simulink model "FFM_Punch"  (R2017a)
settings: Solver=ode3  StartTime=0.0  StopTime=timesteps  FixedStep=data.SIM.Ts  RelTol=1e-3  EnableMultiTasking=on
values from neighbouring files (symbols this model uses):
  data =     [dakota_config.mat]
  downshift_map = data.TCU.upshift.veh_spd_default    [Simulation_results.m]
  upshift_map = data.TCU.upshift.veh_spd_default    [Simulation_results.m]
undefined symbols (not defined in the file or in its folder): air_density, Cd, DiscIntNeverNeededParam, fr_crankshaft, fr_speed_values, g, i_FD, ICE, Low_Ratio, M_Eng_Max, M_Eng_Max_Max, M_Eng_Max_Rpm, mt2m_f, mu_Roll_C0, mu_Roll_C1, mu_Roll_C2, Mv, n_Idle_Eng, Overdrive_Ratio, Re, S_eff_drag, Ts
(part 2 of 15)

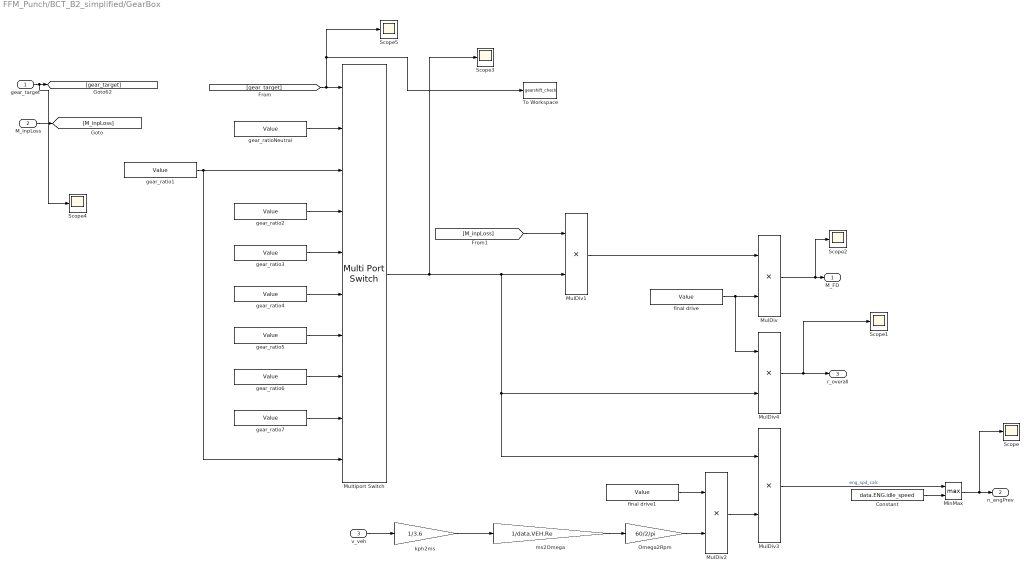
== system FFM_Punch/BCT_B2_simplified/GearBox ==
  gear_target : Inport
  M_inpLoss : Inport  Port=2
  v_veh : Inport  Port=3
  Constant : Constant  Value=data.ENG.idle_speed  OutDataTypeStr=single
  MinMax : MinMax  Function=max  Inputs=2  InputSameDT=on
  MulDiv : Product  Tag=Controls_Lib  Description=MulDiv  Inputs=**  CollapseDim=CollapseDim  OutMin=OutMin  OutMax=OutMax  OutDataTypeStr=single  SampleTime=SampleTime  InputSameDT=on  mask(MulDiv){Inputs=**, Multiplication=Element-wise(.*), CollapseMode=All dimensions, CollapseDim=1, SampleTime=-1, InputSameDT=on, OutMin=[], OutMax=[], OutDataTypeStr=single, LockScale=off, RndMeth=Floor, SaturateOnIntegerOverflow=off}
      mask prompts: Inputs "Number of inputs:"; CollapseMode "Multiply over:"; CollapseDim "Dimension:"; SampleTime "Sample time (-1 for inherited):"; InputSameDT "Require all inputs to have the same data type"; OutMin "Output minimum:"; OutMax "Output maximum:"; OutDataTypeStr "Output data type:"; LockScale "Lock output data type setting against changes by the fixed-point tools"; RndMeth "Integer rounding mode:"; SaturateOnIntegerOverflow "Saturate on integer overflow"
      mask help:
      | Multiply or divide inputs element-wise. Specify one of the following:
      |  a) * or / for each input port. For example, **/* performs the operation 'u1*u2/u3*u4'.
      |  b) scalar specifies the number of input ports to be multiplied.
      | If there is only one input port and the Multiplication parameter is set to Element-wise(.*), a single * or / collapses the input signal using the specified operation.
      mask Help: web([fileparts(which('Lib_built')) filesep 'hlp' filesep 'lib_MulDiv' '.html'], '-helpbrowser')
      mask TypeOptions Inputs: Inputs
      mask TypeOptions Multiplication: Multiplication
      mask TypeOptions CollapseMode: CollapseMode
      mask TypeOptions CollapseDim: CollapseDim
      mask TypeOptions SampleTime: SampleTime
      mask TypeOptions InputSameDT: InputSameDT
      mask TypeOptions OutMin: OutMin
      mask TypeOptions OutMax: OutMax
      mask TypeOptions OutDataTypeStr: OutDataTypeStr
      mask TypeOptions LockScale: LockScale
      mask TypeOptions RndMeth: RndMeth
      mask TypeOptions SaturateOnIntegerOverflow: SaturateOnIntegerOverflow
  MulDiv1 : Product  Tag=Controls_Lib  Description=MulDiv  Inputs=**  CollapseDim=CollapseDim  OutMin=OutMin  OutMax=OutMax  OutDataTypeStr=single  SampleTime=SampleTime  InputSameDT=on  mask(MulDiv){Inputs=**, Multiplication=Element-wise(.*), CollapseMode=All dimensions, CollapseDim=1, SampleTime=-1, InputSameDT=on, OutMin=[], OutMax=[], OutDataTypeStr=single, LockScale=off, RndMeth=Floor, SaturateOnIntegerOverflow=off}
      mask prompts: Inputs "Number of inputs:"; CollapseMode "Multiply over:"; CollapseDim "Dimension:"; SampleTime "Sample time (-1 for inherited):"; InputSameDT "Require all inputs to have the same data type"; OutMin "Output minimum:"; OutMax "Output maximum:"; OutDataTypeStr "Output data type:"; LockScale "Lock output data type setting against changes by the fixed-point tools"; RndMeth "Integer rounding mode:"; SaturateOnIntegerOverflow "Saturate on integer overflow"
      mask help:
      | Multiply or divide inputs element-wise. Specify one of the following:
      |  a) * or / for each input port. For example, **/* performs the operation 'u1*u2/u3*u4'.
      |  b) scalar specifies the number of input ports to be multiplied.
      | If there is only one input port and the Multiplication parameter is set to Element-wise(.*), a single * or / collapses the input signal using the specified operation.
      mask Help: web([fileparts(which('Lib_built')) filesep 'hlp' filesep 'lib_MulDiv' '.html'], '-helpbrowser')
      mask TypeOptions Inputs: Inputs
      mask TypeOptions Multiplication: Multiplication
      mask TypeOptions CollapseMode: CollapseMode
      mask TypeOptions CollapseDim: CollapseDim
      mask TypeOptions SampleTime: SampleTime
      mask TypeOptions InputSameDT: InputSameDT
      mask TypeOptions OutMin: OutMin
      mask TypeOptions OutMax: OutMax
      mask TypeOptions OutDataTypeStr: OutDataTypeStr
      mask TypeOptions LockScale: LockScale
      mask TypeOptions RndMeth: RndMeth
      mask TypeOptions SaturateOnIntegerOverflow: SaturateOnIntegerOverflow
  MulDiv2 : Product  Tag=Controls_Lib  Description=MulDiv  Inputs=**  CollapseDim=CollapseDim  OutMin=OutMin  OutMax=OutMax  OutDataTypeStr=single  SampleTime=SampleTime  InputSameDT=on  mask(MulDiv){Inputs=**, Multiplication=Element-wise(.*), CollapseMode=All dimensions, CollapseDim=1, SampleTime=-1, InputSameDT=on, OutMin=[], OutMax=[], OutDataTypeStr=single, LockScale=off, RndMeth=Floor, SaturateOnIntegerOverflow=off}
      mask prompts: Inputs "Number of inputs:"; CollapseMode "Multiply over:"; CollapseDim "Dimension:"; SampleTime "Sample time (-1 for inherited):"; InputSameDT "Require all inputs to have the same data type"; OutMin "Output minimum:"; OutMax "Output maximum:"; OutDataTypeStr "Output data type:"; LockScale "Lock output data type setting against changes by the fixed-point tools"; RndMeth "Integer rounding mode:"; SaturateOnIntegerOverflow "Saturate on integer overflow"
      mask help:
      | Multiply or divide inputs element-wise. Specify one of the following:
      |  a) * or / for each input port. For example, **/* performs the operation 'u1*u2/u3*u4'.
      |  b) scalar specifies the number of input ports to be multiplied.
      | If there is only one input port and the Multiplication parameter is set to Element-wise(.*), a single * or / collapses the input signal using the specified operation.
      mask Help: web([fileparts(which('Lib_built')) filesep 'hlp' filesep 'lib_MulDiv' '.html'], '-helpbrowser')
      mask TypeOptions Inputs: Inputs
      mask TypeOptions Multiplication: Multiplication
      mask TypeOptions CollapseMode: CollapseMode
      mask TypeOptions CollapseDim: CollapseDim
      mask TypeOptions SampleTime: SampleTime
      mask TypeOptions InputSameDT: InputSameDT
      mask TypeOptions OutMin: OutMin
      mask TypeOptions OutMax: OutMax
      mask TypeOptions OutDataTypeStr: OutDataTypeStr
      mask TypeOptions LockScale: LockScale
      mask TypeOptions RndMeth: RndMeth
      mask TypeOptions SaturateOnIntegerOverflow: SaturateOnIntegerOverflow
  MulDiv3 : Product  Tag=Controls_Lib  Description=MulDiv  Inputs=**  CollapseDim=CollapseDim  OutMin=OutMin  OutMax=OutMax  OutDataTypeStr=single  SampleTime=SampleTime  InputSameDT=on  mask(MulDiv){Inputs=**, Multiplication=Element-wise(.*), CollapseMode=All dimensions, CollapseDim=1, SampleTime=-1, InputSameDT=on, OutMin=[], OutMax=[], OutDataTypeStr=single, LockScale=off, RndMeth=Floor, SaturateOnIntegerOverflow=off}
      mask prompts: Inputs "Number of inputs:"; CollapseMode "Multiply over:"; CollapseDim "Dimension:"; SampleTime "Sample time (-1 for inherited):"; InputSameDT "Require all inputs to have the same data type"; OutMin "Output minimum:"; OutMax "Output maximum:"; OutDataTypeStr "Output data type:"; LockScale "Lock output data type setting against changes by the fixed-point tools"; RndMeth "Integer rounding mode:"; SaturateOnIntegerOverflow "Saturate on integer overflow"
      mask help:
      | Multiply or divide inputs element-wise. Specify one of the following:
      |  a) * or / for each input port. For example, **/* performs the operation 'u1*u2/u3*u4'.
      |  b) scalar specifies the number of input ports to be multiplied.
      | If there is only one input port and the Multiplication parameter is set to Element-wise(.*), a single * or / collapses the input signal using the specified operation.
      mask Help: web([fileparts(which('Lib_built')) filesep 'hlp' filesep 'lib_MulDiv' '.html'], '-helpbrowser')
      mask TypeOptions Inputs: Inputs
      mask TypeOptions Multiplication: Multiplication
      mask TypeOptions CollapseMode: CollapseMode
      mask TypeOptions CollapseDim: CollapseDim
      mask TypeOptions SampleTime: SampleTime
      mask TypeOptions InputSameDT: InputSameDT
      mask TypeOptions OutMin: OutMin
      mask TypeOptions OutMax: OutMax
      mask TypeOptions OutDataTypeStr: OutDataTypeStr
      mask TypeOptions LockScale: LockScale
      mask TypeOptions RndMeth: RndMeth
      mask TypeOptions SaturateOnIntegerOverflow: SaturateOnIntegerOverflow
  MulDiv4 : Product  Tag=Controls_Lib  Description=MulDiv  Inputs=**  CollapseDim=CollapseDim  OutMin=OutMin  OutMax=OutMax  OutDataTypeStr=single  SampleTime=SampleTime  InputSameDT=on  mask(MulDiv){Inputs=**, Multiplication=Element-wise(.*), CollapseMode=All dimensions, CollapseDim=1, SampleTime=-1, InputSameDT=on, OutMin=[], OutMax=[], OutDataTypeStr=single, LockScale=off, RndMeth=Floor, SaturateOnIntegerOverflow=off}
      mask prompts: Inputs "Number of inputs:"; CollapseMode "Multiply over:"; CollapseDim "Dimension:"; SampleTime "Sample time (-1 for inherited):"; InputSameDT "Require all inputs to have the same data type"; OutMin "Output minimum:"; OutMax "Output maximum:"; OutDataTypeStr "Output data type:"; LockScale "Lock output data type setting against changes by the fixed-point tools"; RndMeth "Integer rounding mode:"; SaturateOnIntegerOverflow "Saturate on integer overflow"
      mask help:
      | Multiply or divide inputs element-wise. Specify one of the following:
      |  a) * or / for each input port. For example, **/* performs the operation 'u1*u2/u3*u4'.
      |  b) scalar specifies the number of input ports to be multiplied.
      | If there is only one input port and the Multiplication parameter is set to Element-wise(.*), a single * or / collapses the input signal using the specified operation.
      mask Help: web([fileparts(which('Lib_built')) filesep 'hlp' filesep 'lib_MulDiv' '.html'], '-helpbrowser')
      mask TypeOptions Inputs: Inputs
      mask TypeOptions Multiplication: Multiplication
      mask TypeOptions CollapseMode: CollapseMode
      mask TypeOptions CollapseDim: CollapseDim
      mask TypeOptions SampleTime: SampleTime
      mask TypeOptions InputSameDT: InputSameDT
      mask TypeOptions OutMin: OutMin
      mask TypeOptions OutMax: OutMax
      mask TypeOptions OutDataTypeStr: OutDataTypeStr
      mask TypeOptions LockScale: LockScale
      mask TypeOptions RndMeth: RndMeth
      mask TypeOptions SaturateOnIntegerOverflow: SaturateOnIntegerOverflow
  Multiport Switch : MultiPortSwitch  DataPortOrder=Specify indices  DataPortIndices={0,1,2,3,4,5,6,7}  DataPortForDefault=Additional data port  DiagnosticForDefault=None
  Omega2Rpm : Gain  Gain=60/2/pi
  Scope{,1..5} (6 alike) : Scope
  To Workspace : ToWorkspace  VariableName=gearshift_check  SampleTime=-1
  final drive : Constant  Tag=Controls_Lib  Description=constant  Value=Value  OutMin=OutMin  OutMax=OutMax  OutDataTypeStr=Inherit: Inherit via back propagation  SampleTime=SampleTime  FramePeriod=FramePeriod  mask(Constant){Value=data.DCT.ratio.r_fd, VectorParams1D=on, SampleTime=-1, FramePeriod=inf, OutMin=[], OutMax=[], OutDataTypeStr=Inherit: Inherit via back propagation, LockScale=off}
      mask prompts: Value "Simulink:blkprm_prompts:ConstConstValue"; VectorParams1D "Simulink:blkprm_prompts:AllSrcsVector1D"; SampleTime "Simulink:blkprm_prompts:AllSrcBlksSampleTime"; FramePeriod "Simulink:blkprm_prompts:AllSrcBlksFramePeriod"; OutMin "Simulink:blkprm_prompts:OutputDesignMin"; OutMax "Simulink:blkprm_prompts:OutputDesignMax"; OutDataTypeStr "Simulink:blkprm_prompts:OUTPUT_UNIFIEDDATATYPE"; LockScale "Simulink:blkprm_prompts:LockScale"
      mask help: Output the constant specified by the 'Constant value' parameter.
      mask Help: web([fileparts(which('Lib_built')) filesep 'hlp' filesep 'lib_constant' '.html'], '-helpbrowser')
      mask TypeOptions Value: Value
      mask TypeOptions VectorParams1D: VectorParams1D
      mask TypeOptions SampleTime: SampleTime
      mask TypeOptions FramePeriod: FramePeriod
      mask TypeOptions OutMin: OutMin
      mask TypeOptions OutMax: OutMax
      mask TypeOptions OutDataTypeStr: OutDataTypeStr
      mask TypeOptions LockScale: LockScale
      mask DialogControl ParameterTabVar0 Prompt: Main
      mask Display: disp(get_param(gcb,'Value'))
  final drive1 : Constant  Tag=Controls_Lib  Description=constant  Value=Value  OutMin=OutMin  OutMax=OutMax  OutDataTypeStr=Inherit: Inherit via back propagation  SampleTime=SampleTime  FramePeriod=FramePeriod  mask(Constant){Value=data.DCT.ratio.r_fd, VectorParams1D=on, SampleTime=-1, FramePeriod=inf, OutMin=[], OutMax=[], OutDataTypeStr=Inherit: Inherit via back propagation, LockScale=off}
      mask prompts: Value "Simulink:blkprm_prompts:ConstConstValue"; VectorParams1D "Simulink:blkprm_prompts:AllSrcsVector1D"; SampleTime "Simulink:blkprm_prompts:AllSrcBlksSampleTime"; FramePeriod "Simulink:blkprm_prompts:AllSrcBlksFramePeriod"; OutMin "Simulink:blkprm_prompts:OutputDesignMin"; OutMax "Simulink:blkprm_prompts:OutputDesignMax"; OutDataTypeStr "Simulink:blkprm_prompts:OUTPUT_UNIFIEDDATATYPE"; LockScale "Simulink:blkprm_prompts:LockScale"
      mask help: Output the constant specified by the 'Constant value' parameter.
      mask Help: web([fileparts(which('Lib_built')) filesep 'hlp' filesep 'lib_constant' '.html'], '-helpbrowser')
      mask TypeOptions Value: Value
      mask TypeOptions VectorParams1D: VectorParams1D
      mask TypeOptions SampleTime: SampleTime
      mask TypeOptions FramePeriod: FramePeriod
      mask TypeOptions OutMin: OutMin
      mask TypeOptions OutMax: OutMax
      mask TypeOptions OutDataTypeStr: OutDataTypeStr
      mask TypeOptions LockScale: LockScale
      mask DialogControl ParameterTabVar0 Prompt: Main
      mask Display: disp(get_param(gcb,'Value'))
  gear_ratio1 : Constant  Tag=Controls_Lib  Description=constant  Value=Value  OutMin=OutMin  OutMax=OutMax  OutDataTypeStr=Inherit: Inherit via back propagation  SampleTime=SampleTime  FramePeriod=FramePeriod  mask(Constant){Value=data.DCT.ratio.r_1_C, VectorParams1D=on, SampleTime=-1, FramePeriod=inf, OutMin=[], OutMax=[], OutDataTypeStr=Inherit: Inherit via back propagation, LockScale=off}
      mask prompts: Value "Simulink:blkprm_prompts:ConstConstValue"; VectorParams1D "Simulink:blkprm_prompts:AllSrcsVector1D"; SampleTime "Simulink:blkprm_prompts:AllSrcBlksSampleTime"; FramePeriod "Simulink:blkprm_prompts:AllSrcBlksFramePeriod"; OutMin "Simulink:blkprm_prompts:OutputDesignMin"; OutMax "Simulink:blkprm_prompts:OutputDesignMax"; OutDataTypeStr "Simulink:blkprm_prompts:OUTPUT_UNIFIEDDATATYPE"; LockScale "Simulink:blkprm_prompts:LockScale"
      mask help: Output the constant specified by the 'Constant value' parameter.
      mask Help: web([fileparts(which('Lib_built')) filesep 'hlp' filesep 'lib_constant' '.html'], '-helpbrowser')
      mask TypeOptions Value: Value
      mask TypeOptions VectorParams1D: VectorParams1D
      mask TypeOptions SampleTime: SampleTime
      mask TypeOptions FramePeriod: FramePeriod
      mask TypeOptions OutMin: OutMin
      mask TypeOptions OutMax: OutMax
      mask TypeOptions OutDataTypeStr: OutDataTypeStr
      mask TypeOptions LockScale: LockScale
      mask DialogControl ParameterTabVar0 Prompt: Main
      mask Display: disp(get_param(gcb,'Value'))
  gear_ratio2 : Constant  Tag=Controls_Lib  Description=constant  Value=Value  OutMin=OutMin  OutMax=OutMax  OutDataTypeStr=Inherit: Inherit via back propagation  SampleTime=SampleTime  FramePeriod=FramePeriod  mask(Constant){Value=data.DCT.ratio.r_2_C, VectorParams1D=on, SampleTime=-1, FramePeriod=inf, OutMin=[], OutMax=[], OutDataTypeStr=Inherit: Inherit via back propagation, LockScale=off}
      mask prompts: Value "Simulink:blkprm_prompts:ConstConstValue"; VectorParams1D "Simulink:blkprm_prompts:AllSrcsVector1D"; SampleTime "Simulink:blkprm_prompts:AllSrcBlksSampleTime"; FramePeriod "Simulink:blkprm_prompts:AllSrcBlksFramePeriod"; OutMin "Simulink:blkprm_prompts:OutputDesignMin"; OutMax "Simulink:blkprm_prompts:OutputDesignMax"; OutDataTypeStr "Simulink:blkprm_prompts:OUTPUT_UNIFIEDDATATYPE"; LockScale "Simulink:blkprm_prompts:LockScale"
      mask help: Output the constant specified by the 'Constant value' parameter.
      mask Help: web([fileparts(which('Lib_built')) filesep 'hlp' filesep 'lib_constant' '.html'], '-helpbrowser')
      mask TypeOptions Value: Value
      mask TypeOptions VectorParams1D: VectorParams1D
      mask TypeOptions SampleTime: SampleTime
      mask TypeOptions FramePeriod: FramePeriod
      mask TypeOptions OutMin: OutMin
      mask TypeOptions OutMax: OutMax
      mask TypeOptions OutDataTypeStr: OutDataTypeStr
      mask TypeOptions LockScale: LockScale
      mask DialogControl ParameterTabVar0 Prompt: Main
      mask Display: disp(get_param(gcb,'Value'))
  gear_ratio3 : Constant  Tag=Controls_Lib  Description=constant  Value=Value  OutMin=OutMin  OutMax=OutMax  OutDataTypeStr=Inherit: Inherit via back propagation  SampleTime=SampleTime  FramePeriod=FramePeriod  mask(Constant){Value=data.DCT.ratio.r_3_C, VectorParams1D=on, SampleTime=-1, FramePeriod=inf, OutMin=[], OutMax=[], OutDataTypeStr=Inherit: Inherit via back propagation, LockScale=off}
      mask prompts: Value "Simulink:blkprm_prompts:ConstConstValue"; VectorParams1D "Simulink:blkprm_prompts:AllSrcsVector1D"; SampleTime "Simulink:blkprm_prompts:AllSrcBlksSampleTime"; FramePeriod "Simulink:blkprm_prompts:AllSrcBlksFramePeriod"; OutMin "Simulink:blkprm_prompts:OutputDesignMin"; OutMax "Simulink:blkprm_prompts:OutputDesignMax"; OutDataTypeStr "Simulink:blkprm_prompts:OUTPUT_UNIFIEDDATATYPE"; LockScale "Simulink:blkprm_prompts:LockScale"
      mask help: Output the constant specified by the 'Constant value' parameter.
      mask Help: web([fileparts(which('Lib_built')) filesep 'hlp' filesep 'lib_constant' '.html'], '-helpbrowser')
      mask TypeOptions Value: Value
      mask TypeOptions VectorParams1D: VectorParams1D
      mask TypeOptions SampleTime: SampleTime
      mask TypeOptions FramePeriod: FramePeriod
      mask TypeOptions OutMin: OutMin
      mask TypeOptions OutMax: OutMax
      mask TypeOptions OutDataTypeStr: OutDataTypeStr
      mask TypeOptions LockScale: LockScale
      mask DialogControl ParameterTabVar0 Prompt: Main
      mask Display: disp(get_param(gcb,'Value'))
  gear_ratio4 : Constant  Tag=Controls_Lib  Description=constant  Value=Value  OutMin=OutMin  OutMax=OutMax  OutDataTypeStr=Inherit: Inherit via back propagation  SampleTime=SampleTime  FramePeriod=FramePeriod  mask(Constant){Value=data.DCT.ratio.r_4_C, VectorParams1D=on, SampleTime=-1, FramePeriod=inf, OutMin=[], OutMax=[], OutDataTypeStr=Inherit: Inherit via back propagation, LockScale=off}
      mask prompts: Value "Simulink:blkprm_prompts:ConstConstValue"; VectorParams1D "Simulink:blkprm_prompts:AllSrcsVector1D"; SampleTime "Simulink:blkprm_prompts:AllSrcBlksSampleTime"; FramePeriod "Simulink:blkprm_prompts:AllSrcBlksFramePeriod"; OutMin "Simulink:blkprm_prompts:OutputDesignMin"; OutMax "Simulink:blkprm_prompts:OutputDesignMax"; OutDataTypeStr "Simulink:blkprm_prompts:OUTPUT_UNIFIEDDATATYPE"; LockScale "Simulink:blkprm_prompts:LockScale"
      mask help: Output the constant specified by the 'Constant value' parameter.
      mask Help: web([fileparts(which('Lib_built')) filesep 'hlp' filesep 'lib_constant' '.html'], '-helpbrowser')
      mask TypeOptions Value: Value
      mask TypeOptions VectorParams1D: VectorParams1D
      mask TypeOptions SampleTime: SampleTime
      mask TypeOptions FramePeriod: FramePeriod
      mask TypeOptions OutMin: OutMin
      mask TypeOptions OutMax: OutMax
      mask TypeOptions OutDataTypeStr: OutDataTypeStr
      mask TypeOptions LockScale: LockScale
      mask DialogControl ParameterTabVar0 Prompt: Main
      mask Display: disp(get_param(gcb,'Value'))
  gear_ratio5 : Constant  Tag=Controls_Lib  Description=constant  Value=Value  OutMin=OutMin  OutMax=OutMax  OutDataTypeStr=Inherit: Inherit via back propagation  SampleTime=SampleTime  FramePeriod=FramePeriod  mask(Constant){Value=data.DCT.ratio.r_5_C, VectorParams1D=on, SampleTime=-1, FramePeriod=inf, OutMin=[], OutMax=[], OutDataTypeStr=Inherit: Inherit via back propagation, LockScale=off}
      mask prompts: Value "Simulink:blkprm_prompts:ConstConstValue"; VectorParams1D "Simulink:blkprm_prompts:AllSrcsVector1D"; SampleTime "Simulink:blkprm_prompts:AllSrcBlksSampleTime"; FramePeriod "Simulink:blkprm_prompts:AllSrcBlksFramePeriod"; OutMin "Simulink:blkprm_prompts:OutputDesignMin"; OutMax "Simulink:blkprm_prompts:OutputDesignMax"; OutDataTypeStr "Simulink:blkprm_prompts:OUTPUT_UNIFIEDDATATYPE"; LockScale "Simulink:blkprm_prompts:LockScale"
      mask help: Output the constant specified by the 'Constant value' parameter.
      mask Help: web([fileparts(which('Lib_built')) filesep 'hlp' filesep 'lib_constant' '.html'], '-helpbrowser')
      mask TypeOptions Value: Value
      mask TypeOptions VectorParams1D: VectorParams1D
      mask TypeOptions SampleTime: SampleTime
      mask TypeOptions FramePeriod: FramePeriod
      mask TypeOptions OutMin: OutMin
      mask TypeOptions OutMax: OutMax
      mask TypeOptions OutDataTypeStr: OutDataTypeStr
      mask TypeOptions LockScale: LockScale
      mask DialogControl ParameterTabVar0 Prompt: Main
      mask Display: disp(get_param(gcb,'Value'))
  gear_ratio6 : Constant  Tag=Controls_Lib  Description=constant  Value=Value  OutMin=OutMin  OutMax=OutMax  OutDataTypeStr=Inherit: Inherit via back propagation  SampleTime=SampleTime  FramePeriod=FramePeriod  mask(Constant){Value=data.DCT.ratio.r_6_C, VectorParams1D=on, SampleTime=-1, FramePeriod=inf, OutMin=[], OutMax=[], OutDataTypeStr=Inherit: Inherit via back propagation, LockScale=off}
      mask prompts: Value "Simulink:blkprm_prompts:ConstConstValue"; VectorParams1D "Simulink:blkprm_prompts:AllSrcsVector1D"; SampleTime "Simulink:blkprm_prompts:AllSrcBlksSampleTime"; FramePeriod "Simulink:blkprm_prompts:AllSrcBlksFramePeriod"; OutMin "Simulink:blkprm_prompts:OutputDesignMin"; OutMax "Simulink:blkprm_prompts:OutputDesignMax"; OutDataTypeStr "Simulink:blkprm_prompts:OUTPUT_UNIFIEDDATATYPE"; LockScale "Simulink:blkprm_prompts:LockScale"
      mask help: Output the constant specified by the 'Constant value' parameter.
      mask Help: web([fileparts(which('Lib_built')) filesep 'hlp' filesep 'lib_constant' '.html'], '-helpbrowser')
      mask TypeOptions Value: Value
      mask TypeOptions VectorParams1D: VectorParams1D
      mask TypeOptions SampleTime: SampleTime
      mask TypeOptions FramePeriod: FramePeriod
      mask TypeOptions OutMin: OutMin
      mask TypeOptions OutMax: OutMax
      mask TypeOptions OutDataTypeStr: OutDataTypeStr
      mask TypeOptions LockScale: LockScale
      mask DialogControl ParameterTabVar0 Prompt: Main
      mask Display: disp(get_param(gcb,'Value'))
  gear_ratio7 : Constant  Tag=Controls_Lib  Description=constant  Value=Value  OutMin=OutMin  OutMax=OutMax  OutDataTypeStr=Inherit: Inherit via back propagation  SampleTime=SampleTime  FramePeriod=FramePeriod  mask(Constant){Value=data.DCT.ratio.r_7_C, VectorParams1D=on, SampleTime=-1, FramePeriod=inf, OutMin=[], OutMax=[], OutDataTypeStr=Inherit: Inherit via back propagation, LockScale=off}
      mask prompts: Value "Simulink:blkprm_prompts:ConstConstValue"; VectorParams1D "Simulink:blkprm_prompts:AllSrcsVector1D"; SampleTime "Simulink:blkprm_prompts:AllSrcBlksSampleTime"; FramePeriod "Simulink:blkprm_prompts:AllSrcBlksFramePeriod"; OutMin "Simulink:blkprm_prompts:OutputDesignMin"; OutMax "Simulink:blkprm_prompts:OutputDesignMax"; OutDataTypeStr "Simulink:blkprm_prompts:OUTPUT_UNIFIEDDATATYPE"; LockScale "Simulink:blkprm_prompts:LockScale"
      mask help: Output the constant specified by the 'Constant value' parameter.
      mask Help: web([fileparts(which('Lib_built')) filesep 'hlp' filesep 'lib_constant' '.html'], '-helpbrowser')
      mask TypeOptions Value: Value
      mask TypeOptions VectorParams1D: VectorParams1D
      mask TypeOptions SampleTime: SampleTime
      mask TypeOptions FramePeriod: FramePeriod
      mask TypeOptions OutMin: OutMin
      mask TypeOptions OutMax: OutMax
      mask TypeOptions OutDataTypeStr: OutDataTypeStr
      mask TypeOptions LockScale: LockScale
      mask DialogControl ParameterTabVar0 Prompt: Main
      mask Display: disp(get_param(gcb,'Value'))
  gear_ratioNeutral : Constant  Tag=Controls_Lib  Description=constant  Value=Value  OutMin=OutMin  OutMax=OutMax  OutDataTypeStr=Inherit: Inherit via back propagation  SampleTime=SampleTime  FramePeriod=FramePeriod  mask(Constant){Value=0, VectorParams1D=on, SampleTime=-1, FramePeriod=inf, OutMin=[], OutMax=[], OutDataTypeStr=Inherit: Inherit via back propagation, LockScale=off}
      mask prompts: Value "Simulink:blkprm_prompts:ConstConstValue"; VectorParams1D "Simulink:blkprm_prompts:AllSrcsVector1D"; SampleTime "Simulink:blkprm_prompts:AllSrcBlksSampleTime"; FramePeriod "Simulink:blkprm_prompts:AllSrcBlksFramePeriod"; OutMin "Simulink:blkprm_prompts:OutputDesignMin"; OutMax "Simulink:blkprm_prompts:OutputDesignMax"; OutDataTypeStr "Simulink:blkprm_prompts:OUTPUT_UNIFIEDDATATYPE"; LockScale "Simulink:blkprm_prompts:LockScale"
      mask help: Output the constant specified by the 'Constant value' parameter.
      mask Help: web([fileparts(which('Lib_built')) filesep 'hlp' filesep 'lib_constant' '.html'], '-helpbrowser')
      mask TypeOptions Value: Value
      mask TypeOptions VectorParams1D: VectorParams1D
      mask TypeOptions SampleTime: SampleTime
      mask TypeOptions FramePeriod: FramePeriod
      mask TypeOptions OutMin: OutMin
      mask TypeOptions OutMax: OutMax
      mask TypeOptions OutDataTypeStr: OutDataTypeStr
      mask TypeOptions LockScale: LockScale
      mask DialogControl ParameterTabVar0 Prompt: Main
      mask Display: disp(get_param(gcb,'Value'))
  kph2ms : Gain  Gain=1/3.6
  ms2Omega : Gain  Gain=1/data.VEH.Re  OutDataTypeStr=Inherit: Inherit via back propagation  ParamDataTypeStr=Inherit: Same as input
  M_FD : Outport
  n_engPrev : Outport  Port=2
  r_overall : Outport  Port=3
  wires:
  MulDiv/1 -> Scope2/1, M_FD/1
  gear_target/1 -> Scope4/1, [gear_target]
  [gear_target] -> To Workspace/1, Scope5/1, Multiport Switch/1
  gear_ratio6/1 -> Multiport Switch/8
  gear_ratio5/1 -> Multiport Switch/7
  gear_ratio2/1 -> Multiport Switch/4
  gear_ratio7/1 -> Multiport Switch/9
  gear_ratio1/1 -> Multiport Switch/10, Multiport Switch/3
  gear_ratio4/1 -> Multiport Switch/6
  gear_ratioNeutral/1 -> Multiport Switch/2
  gear_ratio3/1 -> Multiport Switch/5
  M_inpLoss/1 -> [M_inpLoss]
  Multiport Switch/1 -> Scope3/1, MulDiv4/2, MulDiv3/1, MulDiv1/2
  [M_inpLoss] -> MulDiv1/1
  MulDiv1/1 -> MulDiv/1
  final drive/1 -> MulDiv4/1, MulDiv/2
  v_veh/1 -> kph2ms/1
  kph2ms/1 -> ms2Omega/1
  ms2Omega/1 -> Omega2Rpm/1
  Omega2Rpm/1 -> MulDiv2/2
  final drive1/1 -> MulDiv2/1
  MulDiv2/1 -> MulDiv3/2
  MulDiv4/1 -> Scope1/1, r_overall/1
  MulDiv3/1 -> MinMax/1  "eng_spd_calc"
  MinMax/1 -> Scope/1, n_engPrev/1
  Constant/1 -> MinMax/2

== system FFM_Punch/Controller/F02_03_03_03_Shift_Laws_Determination ==
  Throttle_pedal : Inport
  constant : Constant  Value=[1 2 3 4 5 6 7 8]  OutDataTypeStr=uint8
  constant1 : Constant  Value=[1 2 3 4 5 6 7 8]  OutDataTypeStr=uint8
  ts_v_autoModDownAdpLaw_M2 : Lookup_n-D  BreakpointsForDimension1=data.TCU.downshift.pedal  BreakpointsForDimension2=[1 2 3 4 5 6 7 8]  BreakpointsForDimension1DataTypeStr=single  BreakpointsForDimension2DataTypeStr=uint8  BeginIndexSearchUsingPreviousIndexResult=on  Table=downshift_map  TableDataTypeStr=single  ExtrapMethod=Clip  UseLastTableValue=on  InternalRulePriority=Speed  OutDataTypeStr=single  RndMeth=Simplest
      settings: AttributesFormatString=%<Table>
  ts_v_autoModUpAdpLaw_M2 : Lookup_n-D  BreakpointsForDimension1=data.TCU.upshift.pedal  BreakpointsForDimension2=[1 2 3 4 5 6 7 8]  BreakpointsForDimension1DataTypeStr=single  BreakpointsForDimension2DataTypeStr=uint8  BeginIndexSearchUsingPreviousIndexResult=on  Table=upshift_map  TableDataTypeStr=single  ExtrapMethod=Clip  UseLastTableValue=on  InternalRulePriority=Speed  OutDataTypeStr=single  RndMeth=Simplest
      settings: AttributesFormatString=%<Table>
  ts_v_vectThdAutoModDown : Outport
  ts_v_vectThdAutoModUp : Outport  Port=2
  wires:
  constant1/1 -> ts_v_autoModUpAdpLaw_M2/2
  [Throttle_pedal] -> ts_v_autoModDownAdpLaw_M2/1, ts_v_autoModUpAdpLaw_M2/1
  constant/1 -> ts_v_autoModDownAdpLaw_M2/2
  ts_v_autoModDownAdpLaw_M2/1 -> [ts_v_vectThdAutoModDown]
  ts_v_autoModUpAdpLaw_M2/1 -> [ts_v_vectThdAutoModUp]
  [ts_v_vectThdAutoModDown] -> ts_v_vectThdAutoModDown/1
  [ts_v_vectThdAutoModUp] -> ts_v_vectThdAutoModUp/1
  Throttle_pedal/1 -> [Throttle_pedal]

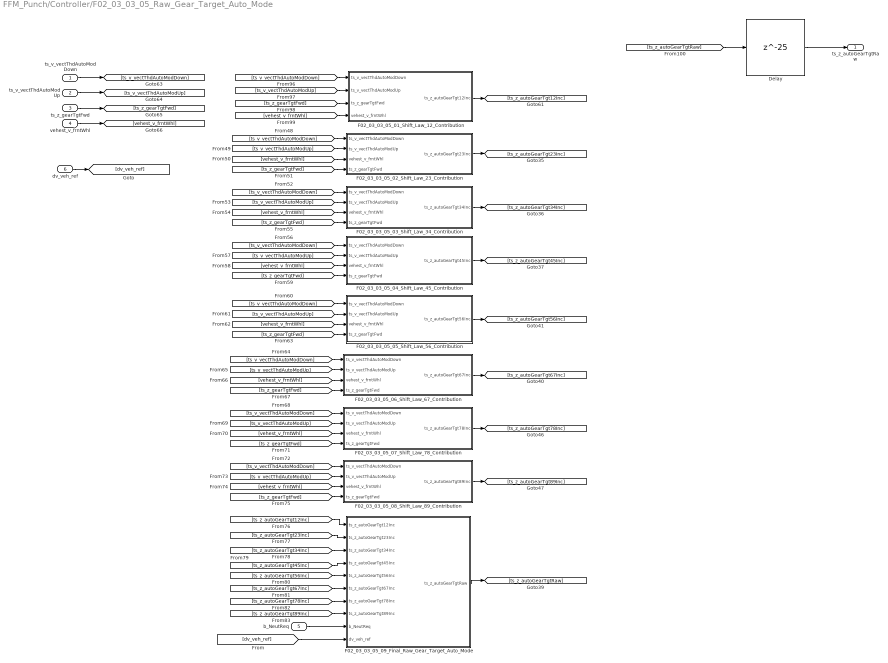
== system FFM_Punch/Controller/F02_03_03_05_Raw_Gear_Target_Auto_Mode ==
  ts_v_vectThdAutoModDown : Inport
  ts_v_vectThdAutoModUp : Inport  Port=2
  ts_z_gearTgtFwd : Inport  Port=3
  vehest_v_frntWhl : Inport  Port=4
  b_NeutReq : Inport  Port=5
  dv_veh_ref : Inport  Tag=Controls_Lib  Description=Inp  Port=6  Interpolate=off
  Delay : Delay  DelayLength=25  InitialCondition=1  UseCircularBuffer=on
  F02_03_03_05_01_Shift_Law_12_Contribution : Subsystem
  F02_03_03_05_02_Shift_Law_23_Contribution : Subsystem
  F02_03_03_05_03_Shift_Law_34_Contribution : Subsystem
  F02_03_03_05_04_Shift_Law_45_Contribution : Subsystem
  F02_03_03_05_05_Shift_Law_56_Contribution : Subsystem
  F02_03_03_05_06_Shift_Law_67_Contribution : Subsystem
  F02_03_03_05_07_Shift_Law_78_Contribution : Subsystem
  F02_03_03_05_08_Shift_Law_89_Contribution : Subsystem
  F02_03_03_05_09_Final_Raw_Gear_Target_Auto_Mode : Subsystem
  ts_z_autoGearTgtRaw : Outport
  wires:
  [ts_z_autoGearTgt89Inc] -> F02_03_03_05_09_Final_Raw_Gear_Target_Auto_Mode/8(ts_z_autoGearTgt89Inc)
  [ts_z_autoGearTgt78Inc] -> F02_03_03_05_09_Final_Raw_Gear_Target_Auto_Mode/7(ts_z_autoGearTgt78Inc)
  [ts_z_autoGearTgt67Inc] -> F02_03_03_05_09_Final_Raw_Gear_Target_Auto_Mode/6(ts_z_autoGearTgt67Inc)
  [ts_z_autoGearTgt56Inc] -> F02_03_03_05_09_Final_Raw_Gear_Target_Auto_Mode/5(ts_z_autoGearTgt56Inc)
  [ts_z_autoGearTgt45Inc] -> F02_03_03_05_09_Final_Raw_Gear_Target_Auto_Mode/4(ts_z_autoGearTgt45Inc)
  [ts_z_autoGearTgt34Inc] -> F02_03_03_05_09_Final_Raw_Gear_Target_Auto_Mode/3(ts_z_autoGearTgt34Inc)
  [ts_z_autoGearTgt23Inc] -> F02_03_03_05_09_Final_Raw_Gear_Target_Auto_Mode/2(ts_z_autoGearTgt23Inc)
  [ts_z_autoGearTgt12Inc] -> F02_03_03_05_09_Final_Raw_Gear_Target_Auto_Mode/1(ts_z_autoGearTgt12Inc)
  F02_03_03_05_08_Shift_Law_89_Contribution/1(ts_z_autoGearTgt89Inc) -> [ts_z_autoGearTgt89Inc]
  [ts_z_gearTgtFwd] -> F02_03_03_05_08_Shift_Law_89_Contribution/4(ts_z_gearTgtFwd)
  [vehest_v_frntWhl] -> F02_03_03_05_08_Shift_Law_89_Contribution/3(vehest_v_frntWhl)
  [ts_v_vectThdAutoModUp] -> F02_03_03_05_08_Shift_Law_89_Contribution/2(ts_v_vectThdAutoModUp)
  [ts_v_vectThdAutoModDown] -> F02_03_03_05_08_Shift_Law_89_Contribution/1(ts_v_vectThdAutoModDown)
  F02_03_03_05_07_Shift_Law_78_Contribution/1(ts_z_autoGearTgt78Inc) -> [ts_z_autoGearTgt78Inc]
  [ts_z_gearTgtFwd] -> F02_03_03_05_07_Shift_Law_78_Contribution/4(ts_z_gearTgtFwd)
  [vehest_v_frntWhl] -> F02_03_03_05_07_Shift_Law_78_Contribution/3(vehest_v_frntWhl)
  [ts_v_vectThdAutoModUp] -> F02_03_03_05_07_Shift_Law_78_Contribution/2(ts_v_vectThdAutoModUp)
  [ts_v_vectThdAutoModDown] -> F02_03_03_05_07_Shift_Law_78_Contribution/1(ts_v_vectThdAutoModDown)
  [ts_z_gearTgtFwd] -> F02_03_03_05_06_Shift_Law_67_Contribution/4(ts_z_gearTgtFwd)
  [vehest_v_frntWhl] -> F02_03_03_05_06_Shift_Law_67_Contribution/3(vehest_v_frntWhl)
  [ts_v_vectThdAutoModUp] -> F02_03_03_05_06_Shift_Law_67_Contribution/2(ts_v_vectThdAutoModUp)
  [ts_v_vectThdAutoModDown] -> F02_03_03_05_06_Shift_Law_67_Contribution/1(ts_v_vectThdAutoModDown)
  [ts_z_gearTgtFwd] -> F02_03_03_05_05_Shift_Law_56_Contribution/4(ts_z_gearTgtFwd)
  [vehest_v_frntWhl] -> F02_03_03_05_05_Shift_Law_56_Contribution/3(vehest_v_frntWhl)
  [ts_v_vectThdAutoModUp] -> F02_03_03_05_05_Shift_Law_56_Contribution/2(ts_v_vectThdAutoModUp)
  [ts_v_vectThdAutoModDown] -> F02_03_03_05_05_Shift_Law_56_Contribution/1(ts_v_vectThdAutoModDown)
  [ts_z_gearTgtFwd] -> F02_03_03_05_04_Shift_Law_45_Contribution/4(ts_z_gearTgtFwd)
  [vehest_v_frntWhl] -> F02_03_03_05_04_Shift_Law_45_Contribution/3(vehest_v_frntWhl)
  [ts_v_vectThdAutoModUp] -> F02_03_03_05_04_Shift_Law_45_Contribution/2(ts_v_vectThdAutoModUp)
  [ts_v_vectThdAutoModDown] -> F02_03_03_05_04_Shift_Law_45_Contribution/1(ts_v_vectThdAutoModDown)
  [ts_z_gearTgtFwd] -> F02_03_03_05_03_Shift_Law_34_Contribution/4(ts_z_gearTgtFwd)
  [vehest_v_frntWhl] -> F02_03_03_05_03_Shift_Law_34_Contribution/3(vehest_v_frntWhl)
  [ts_v_vectThdAutoModUp] -> F02_03_03_05_03_Shift_Law_34_Contribution/2(ts_v_vectThdAutoModUp)
  [ts_v_vectThdAutoModDown] -> F02_03_03_05_03_Shift_Law_34_Contribution/1(ts_v_vectThdAutoModDown)
  [ts_z_gearTgtFwd] -> F02_03_03_05_02_Shift_Law_23_Contribution/4(ts_z_gearTgtFwd)
  [vehest_v_frntWhl] -> F02_03_03_05_02_Shift_Law_23_Contribution/3(vehest_v_frntWhl)
  [ts_v_vectThdAutoModUp] -> F02_03_03_05_02_Shift_Law_23_Contribution/2(ts_v_vectThdAutoModUp)
  [ts_v_vectThdAutoModDown] -> F02_03_03_05_02_Shift_Law_23_Contribution/1(ts_v_vectThdAutoModDown)
  F02_03_03_05_02_Shift_Law_23_Contribution/1(ts_z_autoGearTgt23Inc) -> [ts_z_autoGearTgt23Inc]
  F02_03_03_05_03_Shift_Law_34_Contribution/1(ts_z_autoGearTgt34Inc) -> [ts_z_autoGearTgt34Inc]
  F02_03_03_05_04_Shift_Law_45_Contribution/1(ts_z_autoGearTgt45Inc) -> [ts_z_autoGearTgt45Inc]
  F02_03_03_05_09_Final_Raw_Gear_Target_Auto_Mode/1(ts_z_autoGearTgtRaw) -> [ts_z_autoGearTgtRaw]
  F02_03_03_05_06_Shift_Law_67_Contribution/1(ts_z_autoGearTgt67Inc) -> [ts_z_autoGearTgt67Inc]
  F02_03_03_05_05_Shift_Law_56_Contribution/1(ts_z_autoGearTgt56Inc) -> [ts_z_autoGearTgt56Inc]
  [ts_v_vectThdAutoModDown] -> F02_03_03_05_01_Shift_Law_12_Contribution/1(ts_v_vectThdAutoModDown)
  [ts_v_vectThdAutoModUp] -> F02_03_03_05_01_Shift_Law_12_Contribution/2(ts_v_vectThdAutoModUp)
  [ts_z_gearTgtFwd] -> F02_03_03_05_01_Shift_Law_12_Contribution/3(ts_z_gearTgtFwd)
  [vehest_v_frntWhl] -> F02_03_03_05_01_Shift_Law_12_Contribution/4(vehest_v_frntWhl)
  F02_03_03_05_01_Shift_Law_12_Contribution/1(ts_z_autoGearTgt12Inc) -> [ts_z_autoGearTgt12Inc]
  [ts_z_autoGearTgtRaw] -> Delay/1
  ts_v_vectThdAutoModDown/1 -> [ts_v_vectThdAutoModDown]
  ts_v_vectThdAutoModUp/1 -> [ts_v_vectThdAutoModUp]
  ts_z_gearTgtFwd/1 -> [ts_z_gearTgtFwd]
  vehest_v_frntWhl/1 -> [vehest_v_frntWhl]
  b_NeutReq/1 -> F02_03_03_05_09_Final_Raw_Gear_Target_Auto_Mode/9(b_NeutReq)
  Delay/1 -> ts_z_autoGearTgtRaw/1
  dv_veh_ref/1 -> [dv_veh_ref]
  [dv_veh_ref] -> F02_03_03_05_09_Final_Raw_Gear_Target_Auto_Mode/10(dv_veh_ref)

== system FFM_Punch/Driver Interface/Compare To Constant3 ==
  u : Inport
  Compare : RelationalOperator  Operator=<  OutDataTypeStr=boolean  ZeroCross=off  RndMeth=Nearest  InputSameDT=on
  Constant : Constant  DisableCoverage=on  Value=const  OutDataTypeStr=Inherit: Inherit via back propagation
  y : Outport
  wires:
  u/1 -> Compare/1
  Constant/1 -> Compare/2
  Compare/1 -> y/1

== system FFM_Punch/Driver Interface/Driver Mode_pedalbased ==
  v_ref : Inport
  v_Veh : Inport  Port=2
  n_Eng : Inport  Port=3
  r_Overall : Inport  Port=4
  F_load : Inport  Port=5
  b_NeutReq : Inport  Port=6  OutDataTypeStr=boolean
  dv_veh : Inport  Port=7
  M_eng_Max : Inport  Port=8
  Driver PID Error Calculation and ffwd : Subsystem
  Final PID Computation : Subsystem
  Final Pedal Coordination : Subsystem
  Terminator : Terminator
  Throttle pedal : Outport
  Driver Brake Request : Outport  Port=2
  dv_veh_ref : Outport  Port=3
  wires:
  b_NeutReq/1 -> [b_NeutReq]
  F_load/1 -> Driver PID Error Calculation and ffwd/3(F_load)
  r_Overall/1 -> [r_Overall]
  n_Eng/1 -> Terminator/1
  v_Veh/1 -> [v_Veh]
  v_ref/1 -> [v_Ref]
  Driver PID Error Calculation and ffwd/2(throttle_ffwd) -> [throttle_ffwd]  "throttle_ffwd"
  [v_Ref] -> Driver PID Error Calculation and ffwd/1(v_Ref)
  [v_Veh] -> Driver PID Error Calculation and ffwd/2(v_Veh)
  Driver PID Error Calculation and ffwd/1(err_drv_PIDvehSpd) -> [err_drv_PIDvehSpd]
  [err_drv_PIDvehSpd] -> Final PID Computation/1("err_drv_PIDvehAcc ")
  Final Pedal Coordination/2(Driver Brake Request) -> Driver Brake Request/1
  Final Pedal Coordination/1(Throttle pedal) -> Throttle pedal/1
  [Driver_Brake_Request_Dcy] -> Final Pedal Coordination/1(Driver_Brake_Request_Dcy)
  [Perc_Throtlle_Driv_Req_Dcy] -> Final Pedal Coordination/2(Perc_Throtlle_Driv_Req_Dcy)
  Final PID Computation/2(Perc_Throtlle_Driv_Req_Dcy) -> [Perc_Throtlle_Driv_Req_Dcy]
  dv_veh/1 -> [dv_veh]
  [dv_veh] -> Driver PID Error Calculation and ffwd/4(dv_veh)
  M_eng_Max/1 -> [M_eng_Max]
  [M_eng_Max] -> Driver PID Error Calculation and ffwd/6(M_eng_Max)
  [r_Overall] -> Driver PID Error Calculation and ffwd/5(r_Overall)
  [throttle_ffwd] -> Final PID Computation/2(throttle_ffwd)
  Final PID Computation/1(Driver_Brake_Request_Dcy) -> [Driver_Brake_Request_Dcy]
  [b_NeutReq] -> Final PID Computation/3(b_NeutReq)
  Driver PID Error Calculation and ffwd/3(dv_veh_ref) -> [dv_veh_ref]
  [dv_veh_ref] -> dv_veh_ref/1

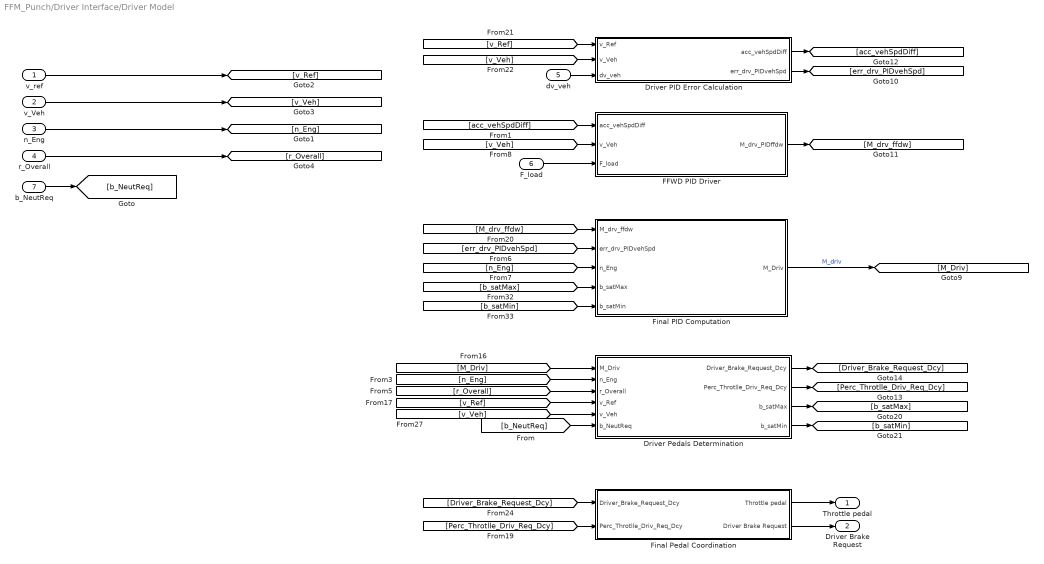
== system FFM_Punch/Driver Interface/Driver Model ==
  v_ref : Inport
  v_Veh : Inport  Port=2
  n_Eng : Inport  Port=3
  r_Overall : Inport  Port=4
  dv_veh : Inport  Port=5
  F_load : Inport  Port=6
  b_NeutReq : Inport  Port=7  OutDataTypeStr=boolean
  Driver PID Error Calculation : Subsystem
  Driver Pedals Determination : Subsystem
  FFWD PID Driver : Subsystem
  Final PID Computation : Subsystem
  Final Pedal Coordination : Subsystem
  Throttle pedal : Outport
  Driver Brake Request : Outport  Port=2
  wires:
  [r_Overall] -> Driver Pedals Determination/3(r_Overall)
  [v_Ref] -> Driver Pedals Determination/4(v_Ref)
  [n_Eng] -> Driver Pedals Determination/2(n_Eng)
  [M_Driv] -> Driver Pedals Determination/1(M_Driv)
  Driver Pedals Determination/2(Perc_Throtlle_Driv_Req_Dcy) -> [Perc_Throtlle_Driv_Req_Dcy]
  Driver Pedals Determination/1(Driver_Brake_Request_Dcy) -> [Driver_Brake_Request_Dcy]
  [Perc_Throtlle_Driv_Req_Dcy] -> Final Pedal Coordination/2(Perc_Throtlle_Driv_Req_Dcy)
  [Driver_Brake_Request_Dcy] -> Final Pedal Coordination/1(Driver_Brake_Request_Dcy)
  Final Pedal Coordination/1(Throttle pedal) -> Throttle pedal/1
  Final Pedal Coordination/2(Driver Brake Request) -> Driver Brake Request/1
  [n_Eng] -> Final PID Computation/3(n_Eng)
  [M_drv_ffdw] -> Final PID Computation/1(M_drv_ffdw)
  [err_drv_PIDvehSpd] -> Final PID Computation/2(err_drv_PIDvehSpd)
  Driver PID Error Calculation/2(err_drv_PIDvehSpd) -> [err_drv_PIDvehSpd]
  Driver PID Error Calculation/1(acc_vehSpdDiff) -> [acc_vehSpdDiff]
  Final PID Computation/1(M_Driv) -> [M_Driv]  "M_driv"
  [v_Veh] -> Driver PID Error Calculation/2(v_Veh)
  [v_Ref] -> Driver PID Error Calculation/1(v_Ref)
  [acc_vehSpdDiff] -> FFWD PID Driver/1(acc_vehSpdDiff)
  FFWD PID Driver/1(M_drv_PIDffdw) -> [M_drv_ffdw]
  [v_Veh] -> FFWD PID Driver/2(v_Veh)
  [v_Veh] -> Driver Pedals Determination/5(v_Veh)
  Driver Pedals Determination/3(b_satMax) -> [b_satMax]
  Driver Pedals Determination/4(b_satMin) -> [b_satMin]
  [b_satMax] -> Final PID Computation/4(b_satMax)
  [b_satMin] -> Final PID Computation/5(b_satMin)
  v_ref/1 -> [v_Ref]
  v_Veh/1 -> [v_Veh]
  n_Eng/1 -> [n_Eng]
  r_Overall/1 -> [r_Overall]
  dv_veh/1 -> Driver PID Error Calculation/3(dv_veh)
  F_load/1 -> FFWD PID Driver/3(F_load)
  b_NeutReq/1 -> [b_NeutReq]
  [b_NeutReq] -> Driver Pedals Determination/6(b_NeutReq)

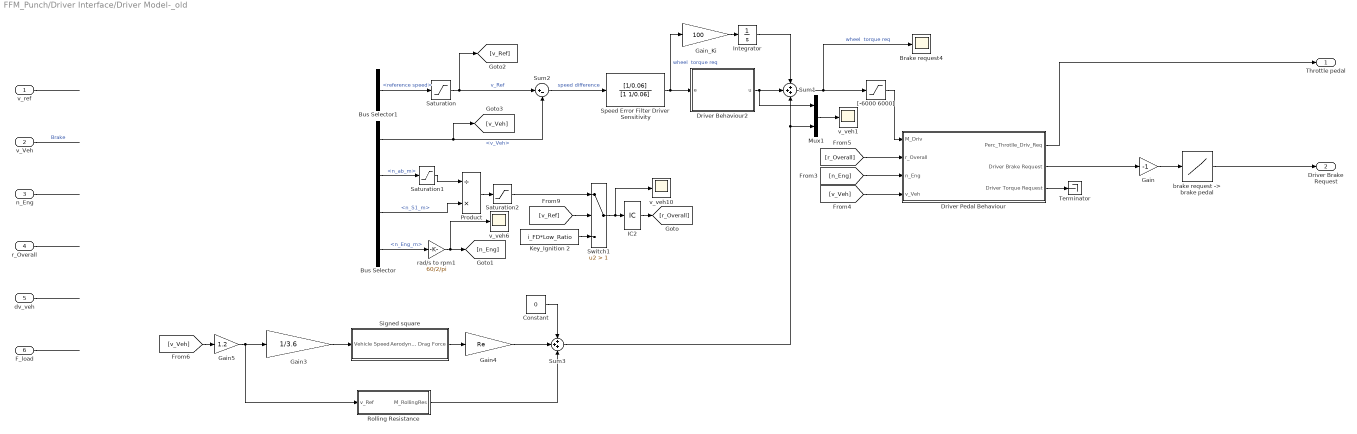
== system FFM_Punch/Driver Interface/Driver Model-_old ==
  v_ref : Inport
  v_Veh : Inport  Port=2
  n_Eng : Inport  Port=3
  r_Overall : Inport  Port=4
  dv_veh : Inport  Port=5
  F_load : Inport  Port=6
  Brake request4 : Scope
  Bus Selector : BusSelector  OutputSignals=v_Veh,n_ab_m,n_S1_m,n_Eng_m
  Bus Selector1 : BusSelector  OutputSignals=reference speed
  Constant : Constant  Value=0
  Driver Behaviour2 : Subsystem  mask(PID Controller){P=Mv*1000/3600*Re*5*0.2*1, I=0, D=3}
      mask prompts: P "Proportional:"; I "Integral:"; D "Derivative:"
      mask help:
      | Enter expressions for proportional, integral, and derivative terms.
      | P+I/s+Ds
      mask Help: This block implements a PID controller where parameters are entered for the Proportional, Integral and Derivative terms. Unmask this block to see how it works. The derivative term is implemented using a true derivative block.
      mask Display: disp('PID')
  Driver Pedal Behaviour : Subsystem
  Gain : Gain  Gain=-1
  Gain3 : Gain  Gain=1/3.6
  Gain4 : Gain  Gain=Re  OutDataTypeStr=Inherit: Inherit via back propagation  ParamDataTypeStr=Inherit: Same as input
  Gain5 : Gain  Gain=1.2
  Gain_Ki : Gain  Gain=100  OutDataTypeStr=Inherit: Inherit via back propagation  ParamDataTypeStr=Inherit: Same as input
  IC2 : InitialCondition  Value=14
  Integrator : Integrator  LimitOutput=on  UpperSaturationLimit=500  LowerSaturationLimit=-500
  Key_Ignition 2 : Constant  Value=i_FD*Low_Ratio
  Mux1 : Mux  Inputs=2
  Product : Product  Inputs=/*  RndMeth=Zero
  Rolling Resistance : Subsystem
  Saturation : Saturate  UpperLimit=inf  LowerLimit=-inf
  Saturation1 : Saturate  UpperLimit=inf  LowerLimit=eps
  Saturation2 : Saturate  UpperLimit=i_FD*Low_Ratio  LowerLimit=i_FD*Overdrive_Ratio
  Signed square : Subsystem
      mask Display: fprintf('Aerodynamics')
  Speed Error Filter Driver Sensitivity : TransferFcn  Numerator=[1/0.06]  Denominator=[1 1/0.06]
  Sum1 : Sum  Inputs=+++
  Sum2 : Sum  Inputs=|+-
  Sum3 : Sum  Inputs=+++
  Switch1 : Switch  Criteria=u2 > Threshold  Threshold=1
  Terminator : Terminator
  "[-6000 6000]" : Saturate  UpperLimit=6000  LowerLimit=-6000
  "brake request -> brake pedal" : Lookup  InputValues=|  Table=|
      InputValues=|
      | [0
      | 
      | 50
      | 
      | 100
      | 
      | 150
      | 
      | 200
      | 
      | 250
      | 
      | 300
      | 
      | 350
      | 
      | 400
      | 
      | 450
      | 
      | 500]
      Table=|
      | [0
      | 
      | 10
      | 
      | 20
      | 
      | 30
      | 
      | 40
      | 
      | 50
      | 
      | 60
      | 
      | 70
      | 
      | 80
      | 
      | 90
      | 
      | 100]
  rad/s to rpm1 : Gain  Gain=60/2/pi
  v_veh1 : Scope
  v_veh10 : Scope
  v_veh6 : Scope
  Throttle pedal : Outport
  Driver Brake Request : Outport  Port=2
  wires:
  Constant/1 -> Sum3/1
  Driver Behaviour2/1(u) -> Sum1/2, Mux1/1
  "brake request -> brake pedal"/1 -> Driver Brake Request/1
  Gain_Ki/1 -> Integrator/1
  Integrator/1 -> Sum1/1
  Gain5/1 -> Rolling Resistance/1(v_Ref), Gain3/1
  IC2/1 -> [r_Overall]
  Key_Ignition 2/1 -> Switch1/3
  [v_Ref] -> Switch1/2
  Switch1/1 -> IC2/1, v_veh10/1
  Saturation/1 -> Sum2/1, [v_Ref]  "v_Ref"
  [v_Veh] -> Gain5/1
  Gain3/1 -> Signed square/1(Vehicle Speed)
  Speed Error Filter Driver Sensitivity/1 -> Driver Behaviour2/1(e), Gain_Ki/1  "wheel  torque req"
  Sum3/1 -> Sum1/3, Mux1/2
  Rolling Resistance/1(M_RollingRes) -> Sum3/3
  Gain4/1 -> Sum3/2
  Signed square/1(Aerodynamic Drag Force) -> Gain4/1
  Mux1/1 -> v_veh1/1
  Bus Selector/3 -> Product/2  "<n_S1_m>"
  Bus Selector/2 -> Saturation1/1  "<n_ab_m>"
  Driver Pedal Behaviour/2(Driver Brake Request) -> Gain/1
  rad/s to rpm1/1 -> v_veh6/1, [n_Eng]
  Bus Selector/4 -> rad/s to rpm1/1  "<n_Eng_m>"
  Saturation1/1 -> Product/1
  Saturation2/1 -> Switch1/1
  Product/1 -> Saturation2/1
  [v_Veh] -> Driver Pedal Behaviour/4(v_Veh)
  Driver Pedal Behaviour/1(Perc_Throtlle_Driv_Req) -> Throttle pedal/1
  [n_Eng] -> Driver Pedal Behaviour/3(n_Eng)
  [r_Overall] -> Driver Pedal Behaviour/2(r_Overall)
  "[-6000 6000]"/1 -> Driver Pedal Behaviour/1(M_Driv)
  Sum1/1 -> "[-6000 6000]"/1, Brake request4/1  "wheel  torque req"
  Gain/1 -> "brake request -> brake pedal"/1
  Sum2/1 -> Speed Error Filter Driver Sensitivity/1  "speed difference"
  Bus Selector1/1 -> Saturation/1  "<reference speed>"
  Bus Selector/1 -> [v_Veh], Sum2/2  "<v_Veh>"
  Driver Pedal Behaviour/3(Driver Torque Request) -> Terminator/1
  r_Overall/1 -> ?
  n_Eng/1 -> ?
  dv_veh/1 -> ?
  F_load/1 -> ?
  v_ref/1 -> ?
  v_Veh/1 -> ?  "Brake"

== system FFM_Punch/ICE/Auxiliaries ==
  Constant : Constant  Value=data.ENG.T_load_auxiliaries
  Gain : Gain  Gain=-1
  M_aux : Outport  Tag=Controls_Lib  Description=Out  InitialOutput=0
  wires:
  Constant/1 -> Gain/1
  Gain/1 -> M_aux/1

== system FFM_Punch/ICE/Friction Torque ==
  ICE Speed : Inport
  Convert : DataTypeConversion  Tag=Controls_Lib  Description=Convert  OutMin=OutMin  OutMax=OutMax  RndMeth=Round  SampleTime=SampleTime  SaturateOnIntegerOverflow=on  mask(Datatype conversion){ConvertRealWorld=Real World Value (RWV), SampleTime=-1, OutMin=[], OutMax=[], OutDataTypeStr=Inherit: Inherit via back propagation, LockScale=off, RndMeth=Round, SaturateOnIntegerOverflow=on}
      mask prompts: ConvertRealWorld "Input and output to have equal:"; SampleTime "Sample time (-1 for inherited):"; OutMin "Output minimum:"; OutMax "Output maximum:"; OutDataTypeStr "Output data type:"; LockScale "Lock output data type setting against changes by the fixed-point tools"; RndMeth "Integer rounding mode:"; SaturateOnIntegerOverflow "Saturate on integer overflow"
      mask help: Convert the input to the data type and scaling of the output.
      mask Help: web([fileparts(which('Lib_built')) filesep 'hlp' filesep 'lib_DataTypeConv' '.html'], '-helpbrowser')
      mask TypeOptions ConvertRealWorld: ConvertRealWorld
      mask TypeOptions SampleTime: SampleTime
      mask TypeOptions OutMin: OutMin
      mask TypeOptions OutMax: OutMax
      mask TypeOptions OutDataTypeStr: OutDataTypeStr
      mask TypeOptions LockScale: LockScale
      mask TypeOptions RndMeth: RndMeth
      mask TypeOptions SaturateOnIntegerOverflow: SaturateOnIntegerOverflow
  Gain : Gain  Gain=(2*pi)/60
  Sign Conversion : Gain  Gain=-1
  Speed Dependant Friction : Lookup  InputValues=data.ENG.friction_speed_values_rad  Table=data.ENG.friction_torque_values  LookUpMeth=Interpolation-Use End Values
  M_fric : Outport  Tag=Controls_Lib  Description=Out  InitialOutput=0
  wires:
  Sign Conversion/1 -> M_fric/1
  ICE Speed/1 -> Gain/1
  Speed Dependant Friction/1 -> Sign Conversion/1
  Convert/1 -> Speed Dependant Friction/1
  Gain/1 -> Convert/1
